simulink model "SkywalkerX8_Longitudinal_Linearized_ReducedOrder"  (R2018a)
settings: Solver=FixedStepAuto  StartTime=0.0  StopTime=10.0  FixedStep=0.02  RelTol=1e-3
undefined symbols (not defined in the file): SkywalkerX8
settings Model: Creator=David  LastModifiedBy=David

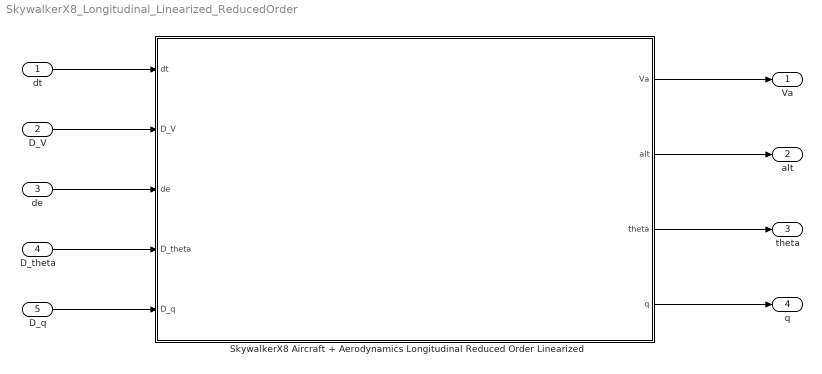
== system SkywalkerX8_Longitudinal_Linearized_ReducedOrder ==
  dt : Inport
  D_V : Inport  Port=2
  de : Inport  Port=3
  D_theta : Inport  Port=4
  D_q : Inport  Port=5
  SkywalkerX8 Aircraft + Aerodynamics Longitudinal Reduced Order Linearized : Subsystem
      mask Display:
      | image('x8SkySunset.png', 'center')
      | 
      | port_label('input', 1, '\delta_t (Unitless)', 'texmode', 'on')
      | port_label('input', 2, 'D_V (m/s)', 'texmode', 'on')
      | port_label('input', 3, '\delta_e (rad)', 'texmode', 'on')
      | port_label('input', 4, 'D_\theta (rad)', 'texmode', 'on')
      | port_label('input', 5, 'D_q (rad/s)', 'texmode', 'on')
      | 
      | 
      | port_label('output', 1, 'V_a (m/s)', 'texmode', 'on')
      | port_label('output', 2, 'Altitude (m)', 'texmode', 'on')
      | port_label('output', 3, '\theta (rad)', 'texmode', 'on')
      | port_label('output', 4, 'q (rad/s)', 'texmode', 'on')
  Va : Outport
  alt : Outport  Port=2
  theta : Outport  Port=3
  q : Outport  Port=4
  wires:
  SkywalkerX8 Aircraft + Aerodynamics Longitudinal Reduced Order Linearized/3(theta) -> theta/1
  SkywalkerX8 Aircraft + Aerodynamics Longitudinal Reduced Order Linearized/1(Va) -> Va/1
  SkywalkerX8 Aircraft + Aerodynamics Longitudinal Reduced Order Linearized/2(alt) -> alt/1
  dt/1 -> SkywalkerX8 Aircraft + Aerodynamics Longitudinal Reduced Order Linearized/1(dt)
  de/1 -> SkywalkerX8 Aircraft + Aerodynamics Longitudinal Reduced Order Linearized/3(de)
  SkywalkerX8 Aircraft + Aerodynamics Longitudinal Reduced Order Linearized/4(q) -> q/1
  D_theta/1 -> SkywalkerX8 Aircraft + Aerodynamics Longitudinal Reduced Order Linearized/4(D_theta)
  D_q/1 -> SkywalkerX8 Aircraft + Aerodynamics Longitudinal Reduced Order Linearized/5(D_q)
  D_V/1 -> SkywalkerX8 Aircraft + Aerodynamics Longitudinal Reduced Order Linearized/2(D_V)

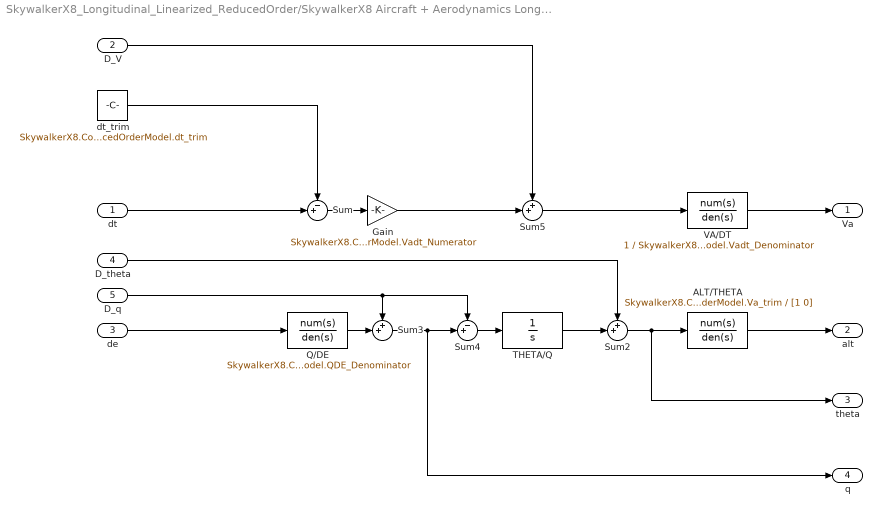
== system SkywalkerX8_Longitudinal_Linearized_ReducedOrder/SkywalkerX8 Aircraft + Aerodynamics Longitudinal Reduced Order Linearized ==
  dt : Inport
  D_V : Inport  Port=2
  de : Inport  Port=3
  D_theta : Inport  Port=4
  D_q : Inport  Port=5
  ALT/THETA : TransferFcn  Numerator=SkywalkerX8.Control.Longitudinal.AlgebraicDesign.ReducedOrderModel.Va_trim  Denominator=[1 0]
  Gain : Gain  Gain=SkywalkerX8.Control.Longitudinal.AlgebraicDesign.ReducedOrderModel.Vadt_Numerator
  Q/DE : TransferFcn  Numerator=SkywalkerX8.Control.Longitudinal.AlgebraicDesign.ReducedOrderModel.QDE_Numerator  Denominator=SkywalkerX8.Control.Longitudinal.AlgebraicDesign.ReducedOrderModel.QDE_Denominator
  Sum : Sum  Inputs=-+|
  Sum2 : Sum  Inputs=++|
  Sum3 : Sum  Inputs=++|
  Sum4 : Sum  Inputs=-+|
  Sum5 : Sum  Inputs=++|
  THETA/Q : TransferFcn  Denominator=[1 0]
  VA/DT : TransferFcn  Numerator=1  Denominator=SkywalkerX8.Control.Longitudinal.AlgebraicDesign.ReducedOrderModel.Vadt_Denominator
  dt_trim : Constant  Value=SkywalkerX8.Control.Longitudinal.AlgebraicDesign.ReducedOrderModel.dt_trim
  Va : Outport
  alt : Outport  Port=2
  theta : Outport  Port=3
  q : Outport  Port=4
  wires:
  de/1 -> Q/DE/1
  ALT/THETA/1 -> alt/1
  Sum2/1 -> theta/1, ALT/THETA/1
  dt/1 -> Sum/2
  VA/DT/1 -> Va/1
  Sum/1 -> Gain/1
  dt_trim/1 -> Sum/1
  THETA/Q/1 -> Sum2/2
  D_theta/1 -> Sum2/1
  Sum3/1 -> q/1, Sum4/2
  Q/DE/1 -> Sum3/2
  Sum4/1 -> THETA/Q/1
  D_q/1 -> Sum4/1, Sum3/1
  Gain/1 -> Sum5/2
  Sum5/1 -> VA/DT/1
  D_V/1 -> Sum5/1
